simulink model "W_server_ClientServer_Model"  (R2024b)
settings: Solver=FixedStepDiscrete  StartTime=0.0  StopTime=10.0  FixedStep=0.05  RelTol=1e-3
settings Model: Tag=EP_AA_WRAPPER_SERVER  DataDictionary=Wrapper_ClientServer_Model.sldd  Creator=yatishc  LastModifiedBy=yatishc
settings OptimizationCC: DefaultParameterBehavior=Inlined  EnhancedBackFolding=on  PassReuseOutputArgsAs=Individual arguments  ZeroExternalMemoryAtStartup=off  ZeroInternalMemoryAtStartup=off  OptimizeBlockOrder=speed  DifferentSizesBufferReuse=on  OptimizationCustomize=off  EfficientTunableParamExpr=on
settings DebuggingCC: ParameterTunabilityLossMsg=error
settings SFSimCC: SimGenImportedTypeDefs=on  MATLABDynamicMemAlloc=off  SimTargetLang=C++
settings RTWCC: Description=Embedded Coder  SystemTargetFile=ert.tlc  GenCodeOnly=on  TemplateMakefile=ert_default_tmf  CustomSourceCode="#include \"ClientServer_Model_adapter.h\""  CustomInitializer=sut_initialize();  DataTypeReplacement=CDataTypesFixedWidth  TargetLang=C++
settings CodeAppCC: ForceParamTrailComments=on  IgnoreCustomStorageClasses=off  MaxIdLength=256  OperatorAnnotations=on  SimulinkDataObjDesc=on  SFDataObjDesc=on  CustomSymbolStrGlobalVar=w_$R$N$M  CustomSymbolStrType=w_$N$R$M_T  InsertBlockDesc=on
settings ERTTargetCC: TargetLangStandard=C++17 (ISO)  GenerateSampleERTMain=on  ERTCustomFileTemplate=example_file_process.tlc  MaxIdInt64=INT64_MAX  MinIdInt64=INT64_MIN  MaxIdUint64=UINT64_MAX  MaxIdInt32=INT32_MAX  MinIdInt32=INT32_MIN  MaxIdUint32=UINT32_MAX  MaxIdInt16=INT16_MAX  MinIdInt16=INT16_MIN  MaxIdUint16=UINT16_MAX  MaxIdInt8=INT8_MAX  MinIdInt8=INT8_MIN  MaxIdUint8=UINT8_MAX

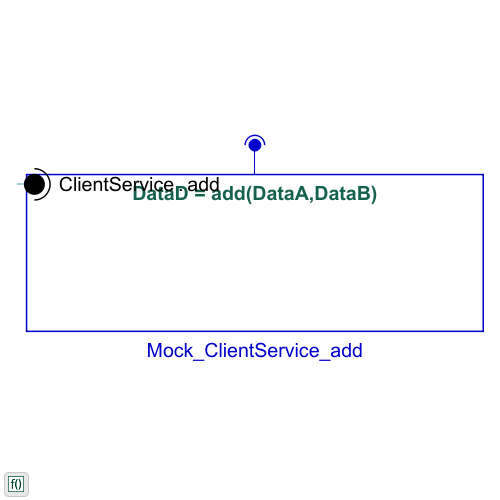
[thumbnail: Simulink's stored preview of the top-level diagram]
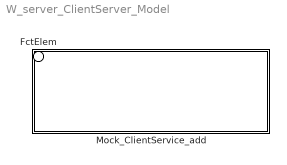
== system W_server_ClientServer_Model ==
  Mock_ClientService_add : Subsystem  TreatAsAtomicUnit=on
  FctElem : Outport  AllowServiceAccess=on  PortName=ClientService  Element=add

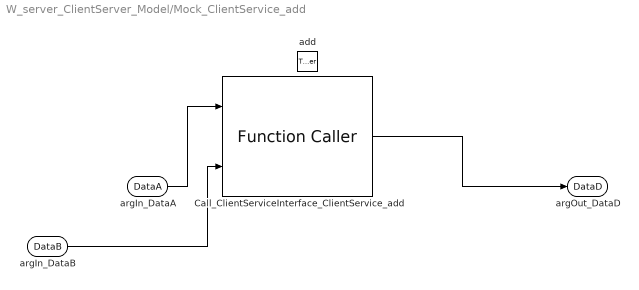
== system W_server_ClientServer_Model/Mock_ClientService_add ==
  add : TriggerPort  TriggerType=function-call  IsSimulinkFunction=on  FunctionName=add  FunctionVisibility=port  ScopeName=ClientService  VariantControl=(inherit)
  Call_ClientServiceInterface_ClientService_add : FunctionCaller  FunctionPrototype=DataD = ClientServiceInterface_ClientService_add(DataA,DataB)  InputArgumentSpecifications=double(0), double(0)  OutputArgumentSpecifications=double(0)
  argIn_DataA : ArgIn  PortDimensions=[1 1]  ArgumentName=DataA
  argIn_DataB : ArgIn  Port=2  PortDimensions=[1 1]  ArgumentName=DataB
  argOut_DataD : ArgOut  PortDimensions=[1 1]  ArgumentName=DataD
  wires:
  argIn_DataA/1 -> Call_ClientServiceInterface_ClientService_add/1
  argIn_DataB/1 -> Call_ClientServiceInterface_ClientService_add/2
  Call_ClientServiceInterface_ClientService_add/1 -> argOut_DataD/1
